simulink model "with_holes"  (R2020b)
settings: Solver=ode23s  StartTime=0.0  StopTime=25  FixedStep=0.2  RelTol=1e-3
PreLoadFcn:
  | sm_tread_drive_param
  | 
  | fuzzy
values from neighbouring files (symbols this model uses):
  ground_x = 12    [sm_tread_drive_param.m]
  ground_y = 10    [sm_tread_drive_param.m]
  tread_l = 2.8    [sm_tread_drive_param.m]
  tread_rad = tread_roller_rad*1.05    (= 0.294)    [sm_tread_drive_param.m]
  tread_roller_rad = tread_h/2*0.8    (= 0.28)    [sm_tread_drive_param.m]
  tread_sep = 1.8    [sm_tread_drive_param.m]
undefined symbols (not defined in the file or in its folder): Extr_Data_RectangleRounded_Holes, floor_d, floor_l, X, Y, Z
libraries: sm_lib x75, nesl_utility x7, Contact_Forces_Lib x6, Parts_Lib x5, fl_lib x4, dspswit3 x1, fuzblock x1, eeGeneralControl x1
(part 1 of 3)
settings Model: Creator=Mario Faragalla  LastModifiedBy=Mario Faragalla
settings DiagnosticsConfigSet: SimMechanicsRigidlyBoundBlock=none

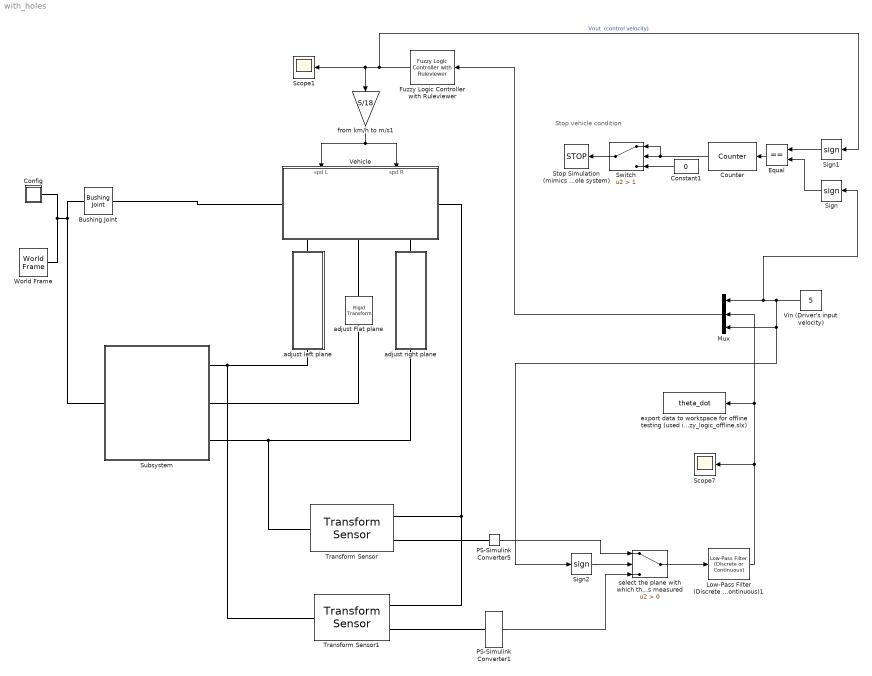
== system with_holes ==
  note: Stop vehicle condition
  Bushing Joint : sm_lib/Joints/Bushing Joint  JointMode=Normal  SenseConstraintForce=off  SenseConstraintForceX=off  SenseConstraintForceY=off  SenseConstraintForceZ=off  SenseConstraintTorque=off  SenseConstraintTorqueX=off  SenseConstraintTorqueY=off  SenseConstraintTorqueZ=off  SenseTotalForce=off  SenseTotalForceX=off  SenseTotalForceY=off  SenseTotalForceZ=off  SenseTotalTorque=off  SenseTotalTorqueX=off  SenseTotalTorqueY=off  SenseTotalTorqueZ=off  CompositeWrenchDir=FollowerOnBase  CompositeWrenchFrame=BaseFrame  PxEquilibriumPosition=0  PxEquilibriumPositionUnits=m  PxSpringStiffness=0  PxSpringStiffnessUnits=N/m  PxDampingCoefficient=0  PxDampingCoefficientUnits=N/(m/s)  PxTorqueActuationMode=NoTorque  PxMotionActuationMode=ComputedMotion  PxSensePosition=off  PxSenseVelocity=off  PxSenseAcceleration=off  PxSenseTorqueForce=off  PxSenseLowerLimitTorqueForce=off  PxSenseUpperLimitTorqueForce=off  PxLowerLimitSpecify=off  PxLowerLimitBound=-1  PxLowerLimitBoundUnits=m  PxLowerLimitStiffness=1e6  PxLowerLimitStiffnessUnits=N/m  PxLowerLimitDamping=1e3  PxLowerLimitDampingUnits=N/(m/s)  PxLowerLimitTransitionRegionWidth=1e-4  PxLowerLimitTransitionRegionWidthUnits=m  PxUpperLimitSpecify=off  PxUpperLimitBound=1  PxUpperLimitBoundUnits=m  PxUpperLimitStiffness=1e6  PxUpperLimitStiffnessUnits=N/m  PxUpperLimitDamping=1e3  PxUpperLimitDampingUnits=N/(m/s)  PxUpperLimitTransitionRegionWidth=1e-4  PxUpperLimitTransitionRegionWidthUnits=m  PxPositionTargetSpecify=on  PxPositionTargetPriority=High  PxPositionTargetValue=-10  PxPositionTargetValueUnits=m  PxVelocityTargetSpecify=off  PxVelocityTargetPriority=High  PxVelocityTargetValue=0  PxVelocityTargetValueUnits=m/s  PyEquilibriumPosition=0  PyEquilibriumPositionUnits=m  PySpringStiffness=0  PySpringStiffnessUnits=N/m  PyDampingCoefficient=0  PyDampingCoefficientUnits=N/(m/s)  PyTorqueActuationMode=NoTorque  PyMotionActuationMode=ComputedMotion  PySensePosition=off  PySenseVelocity=off  PySenseAcceleration=off  PySenseTorqueForce=off  PySenseLowerLimitTorqueForce=off  PySenseUpperLimitTorqueForce=off  PyLowerLimitSpecify=off  PyLowerLimitBound=-1  PyLowerLimitBoundUnits=m  PyLowerLimitStiffness=1e6  PyLowerLimitStiffnessUnits=N/m  PyLowerLimitDamping=1e3  PyLowerLimitDampingUnits=N/(m/s)  PyLowerLimitTransitionRegionWidth=1e-4  PyLowerLimitTransitionRegionWidthUnits=m  PyUpperLimitSpecify=off  PyUpperLimitBound=1  PyUpperLimitBoundUnits=m  PyUpperLimitStiffness=1e6  PyUpperLimitStiffnessUnits=N/m  PyUpperLimitDamping=1e3  PyUpperLimitDampingUnits=N/(m/s)  PyUpperLimitTransitionRegionWidth=1e-4  PyUpperLimitTransitionRegionWidthUnits=m  PyPositionTargetSpecify=on  PyPositionTargetPriority=High  PyPositionTargetValue=0  PyPositionTargetValueUnits=m  PyVelocityTargetSpecify=on  PyVelocityTargetPriority=High  PyVelocityTargetValue=0  PyVelocityTargetValueUnits=m/s  PzEquilibriumPosition=0  PzEquilibriumPositionUnits=m  PzSpringStiffness=0  PzSpringStiffnessUnits=N/m  PzDampingCoefficient=0  PzDampingCoefficientUnits=N/(m/s)  PzTorqueActuationMode=NoTorque  PzMotionActuationMode=ComputedMotion  PzSensePosition=off  PzSenseVelocity=off  PzSenseAcceleration=off  PzSenseTorqueForce=off  PzSenseLowerLimitTorqueForce=off  PzSenseUpperLimitTorqueForce=off  PzLowerLimitSpecify=off  PzLowerLimitBound=-1  PzLowerLimitBoundUnits=m  PzLowerLimitStiffness=1e6  PzLowerLimitStiffnessUnits=N/m  PzLowerLimitDamping=1e3  PzLowerLimitDampingUnits=N/(m/s)  PzLowerLimitTransitionRegionWidth=1e-4  PzLowerLimitTransitionRegionWidthUnits=m  PzUpperLimitSpecify=off  PzUpperLimitBound=1  PzUpperLimitBoundUnits=m  PzUpperLimitStiffness=1e6  PzUpperLimitStiffnessUnits=N/m  PzUpperLimitDamping=1e3  PzUpperLimitDampingUnits=N/(m/s)  PzUpperLimitTransitionRegionWidth=1e-4  PzUpperLimitTransitionRegionWidthUnits=m  PzPositionTargetSpecify=on  PzPositionTargetPriority=High  PzPositionTargetValue=(tread_rad *2)+0.05  PzPositionTargetValueUnits=m  PzVelocityTargetSpecify=off  PzVelocityTargetPriority=High  PzVelocityTargetValue=0  PzVelocityTargetValueUnits=m/s  RxEquilibriumPosition=0  RxEquilibriumPositionUnits=deg  RxSpringStiffness=0  RxSpringStiffnessUnits=N*m/deg  RxDampingCoefficient=0  RxDampingCoefficientUnits=N*m/(deg/s)  RxTorqueActuationMode=NoTorque  RxMotionActuationMode=ComputedMotion  RxSensePosition=off  RxSenseVelocity=off  RxSenseAcceleration=off  RxSenseTorqueForce=off  RxSenseLowerLimitTorqueForce=off  RxSenseUpperLimitTorqueForce=off  RxLowerLimitSpecify=off  RxLowerLimitBound=-90  RxLowerLimitBoundUnits=deg  RxLowerLimitStiffness=1e4  RxLowerLimitStiffnessUnits=N*m/deg  RxLowerLimitDamping=10  RxLowerLimitDampingUnits=N*m/(deg/s)  RxLowerLimitTransitionRegionWidth=0.1  RxLowerLimitTransitionRegionWidthUnits=deg  RxUpperLimitSpecify=off  RxUpperLimitBound=90  RxUpperLimitBoundUnits=deg  RxUpperLimitStiffness=1e4  RxUpperLimitStiffnessUnits=N*m/deg  RxUpperLimitDamping=10  RxUpperLimitDampingUnits=N*m/(deg/s)  RxUpperLimitTransitionRegionWidth=0.1  RxUpperLimitTransitionRegionWidthUnits=deg  RxPositionTargetSpecify=off  RxPositionTargetPriority=High  RxPositionTargetValue=0  RxPositionTargetValueUnits=deg  RxVelocityTargetSpecify=off  RxVelocityTargetPriority=High  RxVelocityTargetValue=0  RxVelocityTargetValueUnits=deg/s  RyEquilibriumPosition=0  RyEquilibriumPositionUnits=deg  RySpringStiffness=0  RySpringStiffnessUnits=N*m/deg  RyDampingCoefficient=0  RyDampingCoefficientUnits=N*m/(deg/s)  RyTorqueActuationMode=NoTorque  RyMotionActuationMode=ComputedMotion  RySensePosition=off  RySenseVelocity=off  RySenseAcceleration=off  RySenseTorqueForce=off  RySenseLowerLimitTorqueForce=off  RySenseUpperLimitTorqueForce=off  RyLowerLimitSpecify=off  RyLowerLimitBound=-90  RyLowerLimitBoundUnits=deg  RyLowerLimitStiffness=1e4  RyLowerLimitStiffnessUnits=N*m/deg  RyLowerLimitDamping=10  RyLowerLimitDampingUnits=N*m/(deg/s)  RyLowerLimitTransitionRegionWidth=0.1  RyLowerLimitTransitionRegionWidthUnits=deg  RyUpperLimitSpecify=off  RyUpperLimitBound=90  RyUpperLimitBoundUnits=deg  RyUpperLimitStiffness=1e4  RyUpperLimitStiffnessUnits=N*m/deg  RyUpperLimitDamping=10  RyUpperLimitDampingUnits=N*m/(deg/s)  RyUpperLimitTransitionRegionWidth=0.1  RyUpperLimitTransitionRegionWidthUnits=deg  RyPositionTargetSpecify=off  RyPositionTargetPriority=High  RyPositionTargetValue=0  RyPositionTargetValueUnits=deg  RyVelocityTargetSpecify=off  RyVelocityTargetPriority=High  RyVelocityTargetValue=0  RyVelocityTargetValueUnits=deg/s  RzEquilibriumPosition=0  RzEquilibriumPositionUnits=deg  RzSpringStiffness=0  RzSpringStiffnessUnits=N*m/deg  RzDampingCoefficient=0  RzDampingCoefficientUnits=N*m/(deg/s)  RzTorqueActuationMode=NoTorque  RzMotionActuationMode=ComputedMotion  RzSensePosition=off  RzSenseVelocity=off  RzSenseAcceleration=off  RzSenseTorqueForce=off  RzSenseLowerLimitTorqueForce=off  RzSenseUpperLimitTorqueForce=off  RzLowerLimitSpecify=off  RzLowerLimitBound=-90  RzLowerLimitBoundUnits=deg  RzLowerLimitStiffness=1e4  RzLowerLimitStiffnessUnits=N*m/deg  RzLowerLimitDamping=10  RzLowerLimitDampingUnits=N*m/(deg/s)  RzLowerLimitTransitionRegionWidth=0.1  RzLowerLimitTransitionRegionWidthUnits=deg  RzUpperLimitSpecify=off  RzUpperLimitBound=90  RzUpperLimitBoundUnits=deg  RzUpperLimitStiffness=1e4  RzUpperLimitStiffnessUnits=N*m/deg  RzUpperLimitDamping=10  RzUpperLimitDampingUnits=N*m/(deg/s)  RzUpperLimitTransitionRegionWidth=0.1  RzUpperLimitTransitionRegionWidthUnits=deg  RzPositionTargetSpecify=off  RzPositionTargetPriority=High  RzPositionTargetValue=0  RzPositionTargetValueUnits=deg  RzVelocityTargetSpecify=off  RzVelocityTargetPriority=High  RzVelocityTargetValue=0  RzVelocityTargetValueUnits=deg/s
  Config : Subsystem
  Constant1 : Constant  Value=0
  Counter : dspswit3/Counter  Direction=Up  CountEvent=Falling edge  CounterSize=User defined  MaxCount=255  InitialCount=0  Output=Count  HitValue=32  ResetInput=off  SamplesPerFrame=1  Ts=1  CntDtype=double  HitDtype=Logical
  Equal : RelationalOperator  Operator===  OutDataTypeStr=boolean  RndMeth=Simplest
  Fuzzy Logic Controller with Ruleviewer : fuzblock/Fuzzy Logic  Controller  with Ruleviewer  fismatrix=fuzzy_pile3  Ts=1
  Low-Pass Filter (Discrete or Continuous)1 : eeGeneralControl/Low-Pass Filter (Discrete or Continuous)  K=10  T=10  B=inf  A=-inf  init_option=Inherited from block input  x0=0  Ts=-1
  Mux : Mux  Inputs=3
  PS-Simulink Converter1 : nesl_utility/PS-Simulink Converter  PhysicalDomain=network_engine_domain  SubClassName=ps_output  LeftPortType=input  RightPortType=output  PseudoPeriodic=off  Frequencies=[]  Unit=inherit  AffineConversion=off
  PS-Simulink Converter5 : nesl_utility/PS-Simulink Converter  PhysicalDomain=network_engine_domain  SubClassName=ps_output  LeftPortType=input  RightPortType=output  PseudoPeriodic=off  Frequencies=[]  Unit=inherit  AffineConversion=off
  Scope1 : Scope
  Scope7 : Scope
  Sign : Signum
  Sign1 : Signum
  Sign2 : Signum
  Stop Simulation (mimics the stop/halt of the whole system) : Stop
  Subsystem : Subsystem
  Switch : Switch  Criteria=u2 > Threshold  Threshold=1  ZeroCross=off
  Transform Sensor : sm_lib/Frames and Transforms/Transform Sensor  MeasurementFrame=Base  SenseAngle=off  SenseAxis=off  SenseAngle1=off  SenseAngle2=off  SenseAngle3=off  SenseQ=off  SenseR=off  SenseOmegaX=off  SenseOmegaY=on  SenseOmegaZ=off  SenseOmega1=off  SenseOmega2=off  SenseOmega3=off  SenseQDot=off  SenseRDot=off  SenseAlphaX=off  SenseAlphaY=off  SenseAlphaZ=off  SenseAlpha1=off  SenseAlpha2=off  SenseAlpha3=off  SenseQDDot=off  SenseRDDot=off  SenseX=off  SenseY=off  SenseZ=off  SenseRad=off  SenseAzim=off  SenseDist=off  SenseInc=off  SenseXDot=off  SenseYDot=off  SenseZDot=off  SenseRadDot=off  SenseAzimDot=off  SenseDistDot=off  SenseIncDot=off  SenseXDDot=off  SenseYDDot=off  SenseZDDot=off  SenseRadDDot=off  SenseAzimDDot=off  SenseDistDDot=off  SenseIncDDot=off
  Transform Sensor1 : sm_lib/Frames and Transforms/Transform Sensor  MeasurementFrame=Base  SenseAngle=off  SenseAxis=off  SenseAngle1=off  SenseAngle2=off  SenseAngle3=off  SenseQ=off  SenseR=off  SenseOmegaX=off  SenseOmegaY=on  SenseOmegaZ=off  SenseOmega1=off  SenseOmega2=off  SenseOmega3=off  SenseQDot=off  SenseRDot=off  SenseAlphaX=off  SenseAlphaY=off  SenseAlphaZ=off  SenseAlpha1=off  SenseAlpha2=off  SenseAlpha3=off  SenseQDDot=off  SenseRDDot=off  SenseX=off  SenseY=off  SenseZ=off  SenseRad=off  SenseAzim=off  SenseDist=off  SenseInc=off  SenseXDot=off  SenseYDot=off  SenseZDot=off  SenseRadDot=off  SenseAzimDot=off  SenseDistDot=off  SenseIncDot=off  SenseXDDot=off  SenseYDDot=off  SenseZDDot=off  SenseRadDDot=off  SenseAzimDDot=off  SenseDistDDot=off  SenseIncDDot=off
  Vehicle : Subsystem
      settings: PortSchema="{\"entries\":[{\"content\":{\"sides\":[{\"content\":{\"connectorIds\":[\"LConn1\"]},\"type\":\"ConnectorPlacement.EquallySpacedRectSide\",\"uuid\":\"fabd707b-f59e-4d45-9dad-4545376ba824\"},{\"content\":{\"connectorIds\":[\"RConn1\"],\"side\":\"RIGHT\"},\"type\":\"ConnectorPlacement.EquallySpacedRectSide\",\"uuid\":\"43ada801-dfb5-4da2-9ab6-aa6db2d15a3d\"},{\"content\":{\"connectorIds\":[\"In1\",\"In2\"],\"side\":\"TOP\"},\"type\":\"ConnectorPlacement.EquallySpacedRectSide\",\"uuid\":\"d91eeb3e-32db-47be-89ab-731665e820f4\"},{\"content\":{\"connectorIds\":[\"RConn2\",\"RConn3\",\"RConn4\"],\"side\":\"BOTTOM\"},\"type\":\"ConnectorPlacement.EquallySpacedRectSide\",\"uuid\":\"76da0d23-ddc9-40dc-a786-2b5b64db7456\"},{\"content\":{\"connectorIds\":[],\"side\":\"HIDDEN\"},\"type\":\"ConnectorPlacement.EquallySpacedRectSide\",\"uuid\":\"48004759-c8c6-47b3-a548-5f1511dff9b7\"}]},\"type\":\"ConnectorPlacement.EquallySpacedConnector\",\"uuid\":\"00c001d2-b8fc-42af-bb12-1d4013db9b0f\"}],\"packageUris\":[\"http://schema.mathworks.com/mf0/Connector/R2020b\"],\"version\":\"1.0\"}"
  Vin (Driver's input velocity) : Constant  Value=5
  World Frame : sm_lib/Frames and Transforms/World Frame
  adjust Flat plane : sm_lib/Frames and Transforms/Rigid Transform  TranslationMethod=StandardAxis  TranslationStandardOffset=(ground_y/4)-0.25  TranslationLengthUnit=m  TranslationStandardAxis=-Y  TranslationCartesianOffset=[0 0 0]  TranslationROffset=0  TranslationROffsetUnits=m  TranslationZOffset=0  TranslationZOffsetUnits=m  TranslationThetaOffset=0  TranslationThetaOffsetUnits=deg  RotationMethod=None  RotationAngleUnits=deg  RotationStandardAxis=+Z  RotationAngle=0.0  RotationArbitraryAxis=[0 0 1]  FollAlignAxisA=+X  BaseAlignAxisA=+Y  FollAlignAxisB=+Y  BaseAlignAxisB=+Z  RotationSequenceAxes=FollowerAxes  RotationSequence=XYX  RotationSequenceAngles=[0 0 0]  RotationSequenceAnglesUnits=deg  RotationMatrix=[1 0 0; 0 1 0; 0 0 1]
  adjust left plane : Subsystem  mask{theta_y=0, offset=up}
      mask prompts: theta_y "Rotation angle"; offset "Direction"
      mask init:
      | switch offset
      |     case 1 %up
      |         offset = -1;
      |     case 2 %down
      |         offset = 1;
      | end
      settings: PortSchema="{\"entries\":[{\"content\":{\"sides\":[{\"content\":{\"connectorIds\":[]},\"type\":\"ConnectorPlacement.EquallySpacedRectSide\",\"uuid\":\"5a52d3ef-8c7d-4b27-92b4-2598d60e8078\"},{\"content\":{\"connectorIds\":[],\"side\":\"RIGHT\"},\"type\":\"ConnectorPlacement.EquallySpacedRectSide\",\"uuid\":\"b8857e3b-9921-4182-868b-79d7343a5054\"},{\"content\":{\"connectorIds\":[\"LConn1\"],\"side\":\"TOP\"},\"type\":\"ConnectorPlacement.EquallySpacedRectSide\",\"uuid\":\"f0e6d2e1-14ee-4037-93b2-310d29a56d19\"},{\"content\":{\"connectorIds\":[\"RConn1\"],\"side\":\"BOTTOM\"},\"type\":\"ConnectorPlacement.EquallySpacedRectSide\",\"uuid\":\"43a24530-94b3-4087-a619-828f9720b0aa\"},{\"content\":{\"connectorIds\":[],\"side\":\"HIDDEN\"},\"type\":\"ConnectorPlacement.EquallySpacedRectSide\",\"uuid\":\"5c2e012c-30d9-4d31-97bb-8e423c4954f3\"}]},\"type\":\"ConnectorPlacement.EquallySpacedConnector\",\"uuid\":\"691960ed-2049-457f-8a6b-8196be0b7b83\"}],\"packageUris\":[\"http://schema.mathworks.com/mf0/Connector/R2020b\"],\"version\":\"1.0\"}"
      mask TypeOptions offset: up | down
  adjust right plane : Subsystem  mask{theta_y=0, offset=down}
      mask prompts: theta_y "Rotation angle"; offset "Direction"
      mask init:
      | switch offset
      |     case 1 %up
      |         offset = 360;
      |     case 2 %down
      |         offset = 2*theta_y;
      | end
      settings: PortSchema="{\"entries\":[{\"content\":{\"sides\":[{\"content\":{\"connectorIds\":[]},\"type\":\"ConnectorPlacement.EquallySpacedRectSide\",\"uuid\":\"5a52d3ef-8c7d-4b27-92b4-2598d60e8078\"},{\"content\":{\"connectorIds\":[],\"side\":\"RIGHT\"},\"type\":\"ConnectorPlacement.EquallySpacedRectSide\",\"uuid\":\"b8857e3b-9921-4182-868b-79d7343a5054\"},{\"content\":{\"connectorIds\":[\"LConn1\"],\"side\":\"TOP\"},\"type\":\"ConnectorPlacement.EquallySpacedRectSide\",\"uuid\":\"f0e6d2e1-14ee-4037-93b2-310d29a56d19\"},{\"content\":{\"connectorIds\":[\"RConn1\"],\"side\":\"BOTTOM\"},\"type\":\"ConnectorPlacement.EquallySpacedRectSide\",\"uuid\":\"43a24530-94b3-4087-a619-828f9720b0aa\"},{\"content\":{\"connectorIds\":[],\"side\":\"HIDDEN\"},\"type\":\"ConnectorPlacement.EquallySpacedRectSide\",\"uuid\":\"5c2e012c-30d9-4d31-97bb-8e423c4954f3\"}]},\"type\":\"ConnectorPlacement.EquallySpacedConnector\",\"uuid\":\"691960ed-2049-457f-8a6b-8196be0b7b83\"}],\"packageUris\":[\"http://schema.mathworks.com/mf0/Connector/R2020b\"],\"version\":\"1.0\"}"
      mask TypeOptions offset: up | down
  export data to workspace for offline testing (used in Test_fuzzy_logic_offline.slx) : ToWorkspace  VariableName=theta_dot  SaveFormat=Timeseries  SampleTime=0.2
  from km/h to m/s1 : Gain  Gain=5/18
  select the plane with which the rotation is measured : Switch  Criteria=u2 > Threshold
  wires:
  from km/h to m/s1/1 -> Vehicle/1(spd L), Vehicle/2(spd R)
  Mux/1 -> Fuzzy Logic Controller with Ruleviewer/1
  Sign/1 -> Equal/2
  Sign1/1 -> Equal/1
  Equal/1 -> Counter/1
  Counter/1 -> Switch/1, Switch/2
  Switch/1 -> Stop Simulation (mimics the stop/halt of the whole system)/1
  Constant1/1 -> Switch/3
  Vin (Driver's input velocity)/1 -> Sign2/1, Mux/3, Mux/1, Sign/1
  Fuzzy Logic Controller with Ruleviewer/1 -> Sign1/1, from km/h to m/s1/1, Scope1/1  "Vout  (control velocity)"
  Sign2/1 -> select the plane with which the rotation is measured/2
  select the plane with which the rotation is measured/1 -> Low-Pass Filter (Discrete or Continuous)1/1
  Low-Pass Filter (Discrete or Continuous)1/1 -> export data to workspace for offline testing (used in Test_fuzzy_logic_offline.slx)/1, Mux/2, Scope7/1
  PS-Simulink Converter5/1 -> select the plane with which the rotation is measured/1
  PS-Simulink Converter1/1 -> select the plane with which the rotation is measured/3
  connections:
  World Frame/RConn1 -- Subsystem/RConn1 -- Bushing Joint/LConn1 -- Config/RConn1
  Vehicle/LConn1 -- Bushing Joint/RConn1
  adjust Flat plane/LConn1 -- Vehicle/RConn3
  Subsystem/LConn1 -- adjust left plane/RConn1 -- Transform Sensor1/LConn1
  Vehicle/RConn1 -- Transform Sensor1/RConn1 -- Transform Sensor/RConn1
  PS-Simulink Converter5/LConn1 -- Transform Sensor/RConn2
  Subsystem/LConn2 -- adjust Flat plane/RConn1
  adjust left plane/LConn1 -- Vehicle/RConn2
  Subsystem/LConn3 -- Transform Sensor/LConn1 -- adjust right plane/RConn1
  adjust right plane/LConn1 -- Vehicle/RConn4
  PS-Simulink Converter1/LConn1 -- Transform Sensor1/RConn2

== system with_holes/Config ==
  Floor : sm_lib/Body Elements/Brick Solid  Commented=on  GraphicAmbientColor=[0.15 0.15 0.15 1.0]  BasedOnType=Density  BrickDimensions=[floor_l floor_l floor_d]  BrickDimensionUnits=m  CenterOfMass=[0 0 0]  CenterOfMassUnits=m  GraphicDiffuseColor=[0.8 0.8 0.8]  Density=1000  DensityUnits=kg/m^3  DoExposeReferenceFrame=on  GraphicEmissiveColor=[0.0 0.0 0.0 1.0]  ExportEntireGeometry=off  SerializedFrames=<Frames><Frame><Id>Frame1</Id><Value><Name>T</Name><Origin><Source>GeometricFeature</Source><FeatureName>+z surface</FeatureName></Origin><PrimaryAxis><DefinedDirection>+Z</DefinedDirection><Source>ReferenceFrame</Source><SourceDirection>+Z</SourceDirection><FeatureName></FeatureName></PrimaryAxis><SecondaryAxis><DefinedDirection>+X</DefinedDirection><Source>ReferenceFrame</Source><SourceDirection>+X</SourceDirection><FeatureName></FeatureName></SecondaryAxis></Value></Frame></Frames>  MarkerShape=Sphere  MarkerSize=10  GraphicType=FromGeometry  InertiaType=CalculateFromGeometry  Mass=1  MassUnits=kg  MomentsOfInertia=[1 1 1]  MomentsOfInertiaUnits=kg*m^2  GraphicOpacity=1.0  ProductsOfInertia=[1 1 1]  ProductsOfInertiaUnits=kg*m^2  GraphicShininess=75  GraphicSpecularColor=[0.5 0.5 0.5 1.0]  GraphicVisPropType=SimpleVisualProperties
  Mechanism Configuration : sm_lib/Utilities/Mechanism Configuration  UniformGravity=Constant  GravityVector=[0 0 -9.80665]  GravityVectorUnits=m/s^2  GravityUnits=m/s^2  LinearizationDelta=0.001  JointModeTransitionNonlinearIterations=2
  Solver Configuration : nesl_utility/Solver Configuration  PhysicalDomain=network_engine_domain  SubClassName=solver  LeftPortType=input  RightPortType=generic  Tones=[]  Harmonics=[]  SimulateNoise=off  Profile=off  UseLocalSampling=off  EnableSwitchedLinearOptims=on  FrequencyDomain=off  UseCCode=off  RelTol=0.001  AbsTol=1e-06  MinStep=1e-09  ToWorkspace=off  RevertToSquareIcSolve=off  NumHomotopyIterations=100  PhasorMode=off  PhasorModeNumHarmonics=1  DoDC=off  ResidualTolerance=1e-09  UseLocalSolver=off  LocalSolverChoice=NE_BACKWARD_EULER_ADVANCER  LocalSolverSampleTime=0.001  DoFixedCost=off  MaxNonlinIter=3  MaxModeIter=2  ComputeImpulses=off  ImpulseIterations=2  LinearAlgebra=Sparse  EquationFormulation=NE_TIME_EF  DelaysMemoryBudget=1024  AutomaticFiltering=on  FilteringTimeConstant=0.001  PartitionStorageMethod=AS_NEEDED  PartitionMemoryBudget=1024  PartitionMethod=FAST
  C : PMIOPort  Side=Right
  connections:
  C/RConn1 -- Floor/LConn1 -- Solver Configuration/RConn1 -- Mechanism Configuration/RConn1

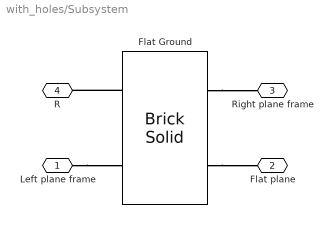
== system with_holes/Subsystem ==
  Flat Ground : sm_lib/Body Elements/Brick Solid  GraphicAmbientColor=[0.15 0.15 0.15 1.0]  BasedOnType=Density  BrickDimensions=[ground_x-3 ground_y 0.5]  BrickDimensionUnits=m  CenterOfMass=[0 0 0]  CenterOfMassUnits=m  GraphicDiffuseColor=[0.5 0.5 0.5]  Density=1000  DensityUnits=kg/m^3  DoExposeReferenceFrame=on  GraphicEmissiveColor=[0.0 0.0 0.0 1.0]  ExportEntireGeometry=off  SerializedFrames=<Frames><Frame><Id>Frame1</Id><Value><Name>F1</Name><Origin><Source>GeometricFeature</Source><FeatureName>-x surface</FeatureName></Origin><PrimaryAxis><DefinedDirection>+Z</DefinedDirection><Source>ReferenceFrame</Source><SourceDirection>+Z</SourceDirection><FeatureName></FeatureName></PrimaryAxis><SecondaryAxis><DefinedDirection>+X</DefinedDirection><Source>ReferenceFrame</Source><SourceDirection>+X</SourceDirection><FeatureName></FeatureName></SecondaryAxis></Value></Frame><Frame><Id>Frame2</Id><Value><Name>Contact F</Name><Origin><Source>CenterOfMassFrame</Source><FeatureName></FeatureName></Origin><PrimaryAxis><DefinedDirection>+Z</DefinedDirection><Source>ReferenceFrame</Source><SourceDirection>+Y</SourceDirection><FeatureName></FeatureName></PrimaryAxis><SecondaryAxis><DefinedDirection>+X</DefinedDirection><Source>ReferenceFrame</Source><SourceDirection>+X</SourceDirection><FeatureName></FeatureName></SecondaryAxis></Value></Frame><Frame><Id>Frame3</Id><Value><Name>F2</Name><Origin><Source>GeometricFeature</Source><FeatureName>+x surface</FeatureName></Origin><PrimaryAxis><DefinedDirection>+Z</DefinedDirection><Source>ReferenceFrame</Source><SourceDirection>+Z</SourceDirection><FeatureName></FeatureName></PrimaryAxis><SecondaryAxis><DefinedDirection>+X</DefinedDirection><Source>ReferenceFrame</Source><SourceDirection>+X</SourceDirection><FeatureName></FeatureName></SecondaryAxis></Value></Frame></Frames>  MarkerShape=Sphere  MarkerSize=10  GraphicType=FromGeometry  InertiaType=CalculateFromGeometry  Mass=1  MassUnits=kg  MomentsOfInertia=[1 1 1]  MomentsOfInertiaUnits=kg*m^2  GraphicOpacity=1.0  ProductsOfInertia=[0 0 0]  ProductsOfInertiaUnits=kg*m^2  GraphicShininess=75  GraphicSpecularColor=[0.5 0.5 0.5 1.0]  GraphicVisPropType=SimpleVisualProperties
  Left plane frame : PMIOPort  Side=Left
  Flat plane : PMIOPort  Port=2  Side=Left
  Right plane frame : PMIOPort  Port=3  Side=Left
  R : PMIOPort  Port=4  Side=Right
  connections:
  Flat Ground/LConn2 -- Flat plane/RConn1
  Flat Ground/RConn1 -- R/RConn1
  Left plane frame/RConn1 -- Flat Ground/RConn2
  Flat Ground/LConn1 -- Right plane frame/RConn1

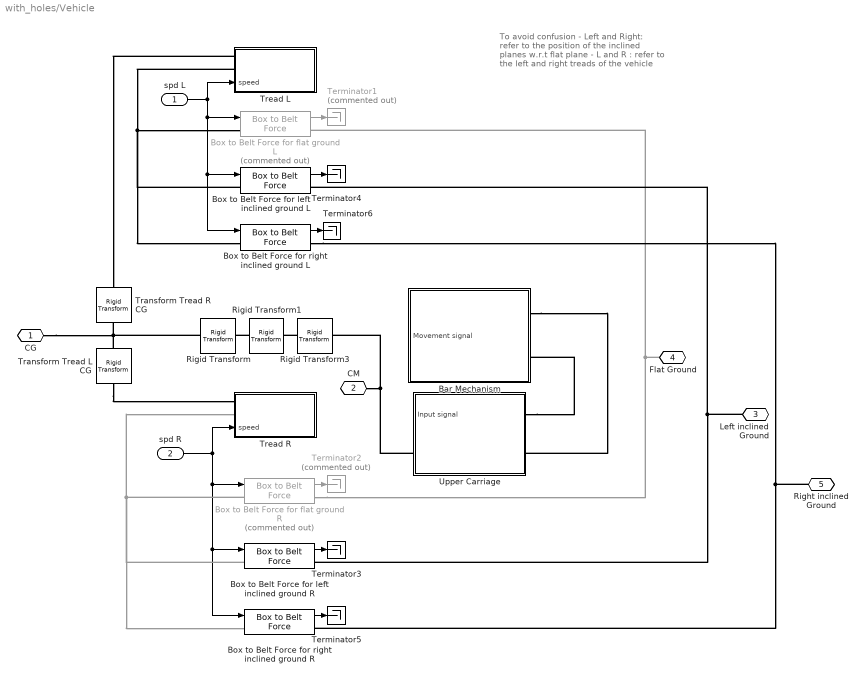
== system with_holes/Vehicle ==
  note: To avoid confusion
      |
      | - Left and Right: refer to the position of the inclined planes w.r.t flat plane
      |
      | - L and R : refer to the left and right treads of the vehicle
  spd L : Inport
  spd R : Inport  Port=2
  Bar Mechanism : Subsystem  mask{barA=3.5, barA1=0.6, trianA=1.2, barB1=1, barB2=0.8, barB3=0.1, barAlpha=80, barA4=0.1, trianR=0.05, barD=0.3, L=0.6, H=0.6, bar_weight=0.8, triangle_weight=1.818, a0=0}
      mask prompts: barA "A1"; barA1 "A2"; trianA "A3"; barB1 "B1"; barB2 "B2"; barB3 "B3"; barAlpha "beta"; barA4 "R1"; trianR "R2"; barD "D"; bar_weight "Bar weight (ton)"; triangle_weight "Triangle weight (ton)"; a0 "alpha"
      mask init:
      | hDistanceBetweenBars = L;
      | vDistanceBetweenBars = H;
      | 
      | barH = (barB1/2-barB2/2)/cosd(barAlpha);
      | barXCoords = [barB1/2,-barB1/2,-barB1/2,-barB1/2+barH*cosd(barAlpha),-barB1/2+barH*cosd(barAlpha),...
      |     barB1/2-barH*cosd(barAlpha),barB1/2-barH*cosd(barAlpha),barB1/2,barB1/2];
      | barYCoords = [barA,barA,barA-barA1,barA-barA1-barH*sind(barAlpha),0,0,barA-barA1-barH*sind(barAlpha),barA-barA1,barA];
      | 
      | barCoords = [barXCoords',barYCoords'];
      | 
      | 
      | barExtraAngle = linspace(0,pi,10);
      | barExtraXCoords = [barD/2,(barD/2)*cos(barExtraAngle),-barD/2];
      | barExtraYCoords = [0,barA1+(barD/2)*sin(barExtraAngle),0];
      | barExtraCoords = [barExtraXCoords',barExtraYCoords'];
      | 
      | 
      | 
      | trianB = sqrt(hDistanceBetweenBars^2+vDistanceBetweenBars^2);
      | %trianA = A;
      | %trianR = 0.05;
      | trianH = sqrt(trianA^2+trianB^2);
      | trianAlpha = 180-atand(trianH/trianR)-atand(trianA/trianB);
      | trianGamma = 90-atand(trianR/trianH)-(90-atand(trianB/trianA));
      | trianXCoords = [trianR*cos(linspace(pi,pi*(3/2),10)),trianB+trianR*cos(linspace(-pi/2,trianAlpha*pi/180,20)),...
      |     trianR*cos(linspace(trianGamma*pi/180,pi,20))];
      |     %,...
      |     %trianR*cos(linspace(pi/3,pi,10))];
      | trianYCoords = [trianR*sin(linspace(pi,pi*(3/2),10)),trianR*sin(linspace(-pi/2,trianAlpha*pi/180,20)),...
      |     trianA+trianR*sin(linspace(trianGamma*pi/180,pi,20))];
      |     %,...
      |     %trianA+trianR*sin(linspace(pi/3,pi,10))];
      | trianCoords = [trianXCoords',trianYCoords'];
      mask DialogControl Container12 Prompt: Dimensions
      mask DialogControl Container11 Prompt: Initial Conditions
      mask Display: image('$imagefile'); % Use "Edit Image" on toolstrip to change.
  Box to Belt Force for flat ground L : Contact_Forces_Lib/2D/Composite Forces/Box to Belt Force  Commented=on  box_l=ground_x-3  box_h=ground_y/2  belt_l=tread_l*1.7  belt_h=(tread_rad+0.1)*2  contact_circle_rad_box2belt=0  force_law_box2belt=Linear  k_contact_box2belt=1e6  b_contact_box2belt=1e5  pen_full_damp_F_box2belt=1e-4  pen_exponent_box2belt=1  friction_law_box2belt=Stick-Slip Continuous  mu_kinetic_box2belt=0.35  mu_static_box2belt=0.4  v_thr_box2belt=0.001  vis_on_box2belt=on  vis_opc_en_box2belt=0  vis_len_boxz=0.1  vis_len_boxx=0.005  vis_len_beltz=0.1  vis_len_beltx=0.005  vis_clr_box2belt=[0 0.2 0.2]  vis_opc_box2belt=0.7
      settings: SourceProductName=Simscape Multibody Contact Forces Library
  Box to Belt Force for flat ground R : Contact_Forces_Lib/2D/Composite Forces/Box to Belt Force  Commented=on  box_l=ground_x-3  box_h=ground_y/2  belt_l=tread_l*1.7  belt_h=(tread_rad+0.1)*2  contact_circle_rad_box2belt=0  force_law_box2belt=Linear  k_contact_box2belt=1e6  b_contact_box2belt=1e5  pen_full_damp_F_box2belt=1e-4  pen_exponent_box2belt=1  friction_law_box2belt=Stick-Slip Continuous  mu_kinetic_box2belt=0.35  mu_static_box2belt=0.4  v_thr_box2belt=0.001  vis_on_box2belt=on  vis_opc_en_box2belt=0  vis_len_boxz=0.1  vis_len_boxx=0.005  vis_len_beltz=0.1  vis_len_beltx=0.005  vis_clr_box2belt=[0 0.2 0.2]  vis_opc_box2belt=0.7
      settings: SourceProductName=Simscape Multibody Contact Forces Library
  Box to Belt Force for left inclined ground L : Contact_Forces_Lib/2D/Composite Forces/Box to Belt Force  box_l=ground_x*2  box_h=ground_y/2  belt_l=tread_l*1.7  belt_h=(tread_rad+0.1)*2  contact_circle_rad_box2belt=0  force_law_box2belt=Linear  k_contact_box2belt=1e6  b_contact_box2belt=1e5  pen_full_damp_F_box2belt=1e-4  pen_exponent_box2belt=1  friction_law_box2belt=Stick-Slip Continuous  mu_kinetic_box2belt=0.35  mu_static_box2belt=0.4  v_thr_box2belt=0.001  vis_on_box2belt=on  vis_opc_en_box2belt=0  vis_len_boxz=0.1  vis_len_boxx=0.005  vis_len_beltz=0.1  vis_len_beltx=0.005  vis_clr_box2belt=[0 0.2 0.2]  vis_opc_box2belt=0.7
      settings: SourceProductName=Simscape Multibody Contact Forces Library
  Box to Belt Force for left inclined ground R : Contact_Forces_Lib/2D/Composite Forces/Box to Belt Force  box_l=ground_x*2  box_h=ground_y/2  belt_l=tread_l*1.7  belt_h=(tread_rad+0.1)*2  contact_circle_rad_box2belt=0  force_law_box2belt=Linear  k_contact_box2belt=1e6  b_contact_box2belt=1e5  pen_full_damp_F_box2belt=1e-4  pen_exponent_box2belt=1  friction_law_box2belt=Stick-Slip Continuous  mu_kinetic_box2belt=0.35  mu_static_box2belt=0.4  v_thr_box2belt=0.001  vis_on_box2belt=on  vis_opc_en_box2belt=0  vis_len_boxz=0.1  vis_len_boxx=0.005  vis_len_beltz=0.1  vis_len_beltx=0.005  vis_clr_box2belt=[0 0.2 0.2]  vis_opc_box2belt=0.7
      settings: SourceProductName=Simscape Multibody Contact Forces Library
  Box to Belt Force for right inclined ground L : Contact_Forces_Lib/2D/Composite Forces/Box to Belt Force  box_l=ground_x*2  box_h=ground_y/2  belt_l=tread_l*1.7  belt_h=(tread_rad+0.1)*2  contact_circle_rad_box2belt=0  force_law_box2belt=Linear  k_contact_box2belt=1e6  b_contact_box2belt=1e5  pen_full_damp_F_box2belt=1e-4  pen_exponent_box2belt=1  friction_law_box2belt=Stick-Slip Continuous  mu_kinetic_box2belt=0.35  mu_static_box2belt=0.4  v_thr_box2belt=0.001  vis_on_box2belt=on  vis_opc_en_box2belt=0  vis_len_boxz=0.1  vis_len_boxx=0.005  vis_len_beltz=0.1  vis_len_beltx=0.005  vis_clr_box2belt=[0 0.2 0.2]  vis_opc_box2belt=0.7
      settings: SourceProductName=Simscape Multibody Contact Forces Library
  Box to Belt Force for right inclined ground R : Contact_Forces_Lib/2D/Composite Forces/Box to Belt Force  box_l=ground_x*2  box_h=ground_y/2  belt_l=tread_l*1.7  belt_h=(tread_rad+0.1)*2  contact_circle_rad_box2belt=0  force_law_box2belt=Linear  k_contact_box2belt=1e6  b_contact_box2belt=1e5  pen_full_damp_F_box2belt=1e-4  pen_exponent_box2belt=1  friction_law_box2belt=Stick-Slip Continuous  mu_kinetic_box2belt=0.35  mu_static_box2belt=0.4  v_thr_box2belt=0.001  vis_on_box2belt=on  vis_opc_en_box2belt=0  vis_len_boxz=0.1  vis_len_boxx=0.005  vis_len_beltz=0.1  vis_len_beltx=0.005  vis_clr_box2belt=[0 0.2 0.2]  vis_opc_box2belt=0.7
      settings: SourceProductName=Simscape Multibody Contact Forces Library
  Rigid Transform : sm_lib/Frames and Transforms/Rigid Transform  TranslationMethod=StandardAxis  TranslationStandardOffset=0.7  TranslationLengthUnit=m  TranslationStandardAxis=-Z  TranslationCartesianOffset=[0 0 0]  TranslationROffset=0  TranslationROffsetUnits=m  TranslationZOffset=0  TranslationZOffsetUnits=m  TranslationThetaOffset=0  TranslationThetaOffsetUnits=deg  RotationMethod=None  RotationAngleUnits=deg  RotationStandardAxis=+Z  RotationAngle=0.0  RotationArbitraryAxis=[0 0 1]  FollAlignAxisA=+X  BaseAlignAxisA=+Y  FollAlignAxisB=+Y  BaseAlignAxisB=+Z  RotationSequenceAxes=FollowerAxes  RotationSequence=XYX  RotationSequenceAngles=[0 0 0]  RotationSequenceAnglesUnits=deg  RotationMatrix=[1 0 0; 0 1 0; 0 0 1]
  Rigid Transform1 : sm_lib/Frames and Transforms/Rigid Transform  TranslationMethod=StandardAxis  TranslationStandardOffset=-2  TranslationLengthUnit=m  TranslationStandardAxis=+X  TranslationCartesianOffset=[0 0 0]  TranslationROffset=0  TranslationROffsetUnits=m  TranslationZOffset=0  TranslationZOffsetUnits=m  TranslationThetaOffset=0  TranslationThetaOffsetUnits=deg  RotationMethod=None  RotationAngleUnits=deg  RotationStandardAxis=+Z  RotationAngle=0.0  RotationArbitraryAxis=[0 0 1]  FollAlignAxisA=+X  BaseAlignAxisA=+Y  FollAlignAxisB=+Y  BaseAlignAxisB=+Z  RotationSequenceAxes=FollowerAxes  RotationSequence=XYX  RotationSequenceAngles=[0 0 0]  RotationSequenceAnglesUnits=deg  RotationMatrix=[1 0 0; 0 1 0; 0 0 1]
  Rigid Transform3 : sm_lib/Frames and Transforms/Rigid Transform  TranslationMethod=StandardAxis  TranslationStandardOffset=0.1  TranslationLengthUnit=m  TranslationStandardAxis=+Y  TranslationCartesianOffset=[0 0 0]  TranslationROffset=0  TranslationROffsetUnits=m  TranslationZOffset=0  TranslationZOffsetUnits=m  TranslationThetaOffset=0  TranslationThetaOffsetUnits=deg  RotationMethod=None  RotationAngleUnits=deg  RotationStandardAxis=+Z  RotationAngle=0.0  RotationArbitraryAxis=[0 0 1]  FollAlignAxisA=+X  BaseAlignAxisA=+Y  FollAlignAxisB=+Y  BaseAlignAxisB=+Z  RotationSequenceAxes=FollowerAxes  RotationSequence=XYX  RotationSequenceAngles=[0 0 0]  RotationSequenceAnglesUnits=deg  RotationMatrix=[1 0 0; 0 1 0; 0 0 1]
  Terminator1 : Terminator  Commented=on
  Terminator2 : Terminator  Commented=on
  Terminator{3..6} (4 alike) : Terminator
  Transform Tread L CG : sm_lib/Frames and Transforms/Rigid Transform  TranslationMethod=StandardAxis  TranslationStandardOffset=tread_sep/2  TranslationLengthUnit=m  TranslationStandardAxis=+Y  TranslationCartesianOffset=[0 0 0]  TranslationROffset=0  TranslationROffsetUnits=m  TranslationZOffset=0  TranslationZOffsetUnits=m  TranslationThetaOffset=0  TranslationThetaOffsetUnits=deg  RotationMethod=None  RotationAngleUnits=deg  RotationStandardAxis=+Z  RotationAngle=0.0  RotationArbitraryAxis=[0 0 1]  FollAlignAxisA=+X  BaseAlignAxisA=+Y  FollAlignAxisB=+Y  BaseAlignAxisB=+Z  RotationSequenceAxes=FollowerAxes  RotationSequence=XYX  RotationSequenceAngles=[0 0 0]  RotationSequenceAnglesUnits=deg  RotationMatrix=[1 0 0; 0 1 0; 0 0 1]
  Transform Tread R CG : sm_lib/Frames and Transforms/Rigid Transform  TranslationMethod=StandardAxis  TranslationStandardOffset=tread_sep/2  TranslationLengthUnit=m  TranslationStandardAxis=+Y  TranslationCartesianOffset=[0 0 0]  TranslationROffset=0  TranslationROffsetUnits=m  TranslationZOffset=0  TranslationZOffsetUnits=m  TranslationThetaOffset=0  TranslationThetaOffsetUnits=deg  RotationMethod=None  RotationAngleUnits=deg  RotationStandardAxis=+Z  RotationAngle=0.0  RotationArbitraryAxis=[0 0 1]  FollAlignAxisA=+X  BaseAlignAxisA=+Y  FollAlignAxisB=+Y  BaseAlignAxisB=+Z  RotationSequenceAxes=FollowerAxes  RotationSequence=XYX  RotationSequenceAngles=[0 0 0]  RotationSequenceAnglesUnits=deg  RotationMatrix=[1 0 0; 0 1 0; 0 0 1]
  Tread L : Subsystem
      settings: PortSchema="{\"entries\":[{\"content\":{\"sides\":[{\"content\":{\"connectorIds\":[]},\"type\":\"ConnectorPlacement.EquallySpacedRectSide\",\"uuid\":\"71f54ac7-1acd-4494-b2ba-36120ebb2448\"},{\"content\":{\"connectorIds\":[\"RConn1\",\"RConn2\",\"In1\"],\"side\":\"RIGHT\"},\"type\":\"ConnectorPlacement.EquallySpacedRectSide\",\"uuid\":\"abfaafc8-7934-4bf8-9c1d-7af05f31c6a7\"},{\"content\":{\"connectorIds\":[],\"side\":\"TOP\"},\"type\":\"ConnectorPlacement.EquallySpacedRectSide\",\"uuid\":\"b5262782-7ab0-48f5-b129-0cdfcd7050d8\"},{\"content\":{\"connectorIds\":[],\"side\":\"BOTTOM\"},\"type\":\"ConnectorPlacement.EquallySpacedRectSide\",\"uuid\":\"5c554a08-2f46-428a-a953-6231f81c923d\"},{\"content\":{\"connectorIds\":[],\"side\":\"HIDDEN\"},\"type\":\"ConnectorPlacement.EquallySpacedRectSide\",\"uuid\":\"0cc664ae-e858-4ab8-8762-0f97b2d06f3c\"}]},\"type\":\"ConnectorPlacement.EquallySpacedConnector\",\"uuid\":\"cf0c008a-5e1f-4cc9-b20e-5a159a9bbf66\"}],\"packageUris\":[\"http://schema.mathworks.com/mf0/Connector/R2020b\"],\"version\":\"1.0\"}"
  Tread R : Subsystem
      settings: PortSchema="{\"entries\":[{\"content\":{\"sides\":[{\"content\":{\"connectorIds\":[]},\"type\":\"ConnectorPlacement.EquallySpacedRectSide\",\"uuid\":\"71f54ac7-1acd-4494-b2ba-36120ebb2448\"},{\"content\":{\"connectorIds\":[\"RConn1\",\"RConn2\",\"In1\"],\"side\":\"RIGHT\"},\"type\":\"ConnectorPlacement.EquallySpacedRectSide\",\"uuid\":\"abfaafc8-7934-4bf8-9c1d-7af05f31c6a7\"},{\"content\":{\"connectorIds\":[],\"side\":\"TOP\"},\"type\":\"ConnectorPlacement.EquallySpacedRectSide\",\"uuid\":\"b5262782-7ab0-48f5-b129-0cdfcd7050d8\"},{\"content\":{\"connectorIds\":[],\"side\":\"HIDDEN\"},\"type\":\"ConnectorPlacement.EquallySpacedRectSide\",\"uuid\":\"0cc664ae-e858-4ab8-8762-0f97b2d06f3c\"}]},\"type\":\"ConnectorPlacement.EquallySpacedConnector\",\"uuid\":\"cf0c008a-5e1f-4cc9-b20e-5a159a9bbf66\"}],\"packageUris\":[\"http://schema.mathworks.com/mf0/Connector/R2020b\"],\"version\":\"1.0\"}"
  Upper Carriage : Subsystem  mask{A1=2.87, A2=2.725, A3=3.5, B1=2.8, B2=1.12, B3=0.81, B4=1.845, B5=2.8/2, C1=2.196, CW=11, CCW=10, H=0.6, L=0.6}
      mask prompts: CW "Car Weight (ton)"; CCW "Counter Weight Weight (ton)"; H "H*"; L "L*"
      mask init:
      | counterWeightLength = B3;
      | carLength = A2+A1-counterWeightLength;
      | carWidth = B1;
      | carCabinLength = A2%carLength*0.6;
      | carCabinWidth = B2 %carWidth*0.4;
      | counterWeightWidth = carWidth;
      | carHeight = C1;
      | counterWeightHeight = carHeight;
      | carBarBackX = B4;
      | hDistanceBetweenBars = L;
      | vDistanceBetweenBars = H;
      | %Extrusion in Y
      | carCoordX = [0,0,-carWidth,-carWidth,-carCabinWidth,-carCabinWidth];
      | carCoordY = [0,carLength,carLength,carCabinLength,carCabinLength,0];
      | %plot(carCoordX,carCoordY)
      | 
      | carCoord = [carCoordX',carCoordY'];
      | 
      | counterWeightCoordX = [0,0,-carWidth,-carWidth];
      | counterWeightCoordY = [0,counterWeightLength,counterWeightLength,0];
      | %plot(counterWeightCoordX,counterWeightCoordY)
      | counterWeightCoord = [counterWeightCoordX',counterWeightCoordY'];
      mask DialogControl Control4 Prompt: Connection with bar mechanism
      mask DialogControl Control3 Prompt: H* and L* have to be the same as H and L in bar mechanism
      mask Display: image('$imagefile'); % Use "Edit Image" on toolstrip to change.
  CG : PMIOPort  Side=Left
  CM : PMIOPort  Port=2  Side=Right
  Left inclined Ground : PMIOPort  Port=3  Side=Right
  Flat Ground : PMIOPort  Port=4  Side=Right
  Right inclined Ground : PMIOPort  Port=5  Side=Right
  wires:
  Box to Belt Force for flat ground L/1 -> Terminator1/1
  spd L/1 -> Box to Belt Force for right inclined ground L/1, Box to Belt Force for left inclined ground L/1, Box to Belt Force for flat ground L/1, Tread L/1(speed)
  spd R/1 -> Tread R/1(speed), Box to Belt Force for right inclined ground R/1, Box to Belt Force for left inclined ground R/1, Box to Belt Force for flat ground R/1
  Box to Belt Force for flat ground R/1 -> Terminator2/1
  Box to Belt Force for left inclined ground R/1 -> Terminator3/1
  Box to Belt Force for left inclined ground L/1 -> Terminator4/1
  Box to Belt Force for right inclined ground R/1 -> Terminator5/1
  Box to Belt Force for right inclined ground L/1 -> Terminator6/1
  connections:
  CG/RConn1 -- Rigid Transform/RConn1 -- Transform Tread L CG/LConn1 -- Transform Tread R CG/RConn1
  Transform Tread L CG/RConn1 -- Tread R/RConn1
  Tread L/RConn1 -- Transform Tread R CG/LConn1
  Rigid Transform1/RConn1 -- Rigid Transform/LConn1
  Upper Carriage/LConn1 -- Rigid Transform3/LConn1 -- CM/RConn1
  Upper Carriage/RConn1 -- Bar Mechanism/RConn2
  Bar Mechanism/RConn1 -- Upper Carriage/RConn2
  Rigid Transform3/RConn1 -- Rigid Transform1/LConn1
  Tread L/RConn2 -- Box to Belt Force for left inclined ground L/LConn1 -- Box to Belt Force for right inclined ground L/LConn1 -- Box to Belt Force for flat ground L/LConn1
  Box to Belt Force for flat ground R/RConn1 -- Box to Belt Force for flat ground L/RConn1 -- Flat Ground/RConn1
  Box to Belt Force for flat ground R/LConn1 -- Box to Belt Force for left inclined ground R/LConn1 -- Box to Belt Force for right inclined ground R/LConn1 -- Tread R/RConn2
  Left inclined Ground/RConn1 -- Box to Belt Force for left inclined ground R/RConn1 -- Box to Belt Force for left inclined ground L/RConn1
  Box to Belt Force for right inclined ground L/RConn1 -- Box to Belt Force for right inclined ground R/RConn1 -- Right inclined Ground/RConn1

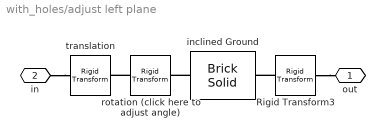
== system with_holes/adjust left plane ==
  Rigid Transform3 : sm_lib/Frames and Transforms/Rigid Transform  TranslationMethod=StandardAxis  TranslationStandardOffset=(ground_y/4)-0.25  TranslationLengthUnit=m  TranslationStandardAxis=+Y  TranslationCartesianOffset=[0 0 0]  TranslationROffset=0  TranslationROffsetUnits=m  TranslationZOffset=0  TranslationZOffsetUnits=m  TranslationThetaOffset=0  TranslationThetaOffsetUnits=deg  RotationMethod=None  RotationAngleUnits=deg  RotationStandardAxis=+Z  RotationAngle=0.0  RotationArbitraryAxis=[0 0 1]  FollAlignAxisA=+X  BaseAlignAxisA=+Y  FollAlignAxisB=+Y  BaseAlignAxisB=+Z  RotationSequenceAxes=FollowerAxes  RotationSequence=XYX  RotationSequenceAngles=[0 0 0]  RotationSequenceAnglesUnits=deg  RotationMatrix=[1 0 0; 0 1 0; 0 0 1]
  inclined Ground : sm_lib/Body Elements/Brick Solid  GraphicAmbientColor=[0.15 0.15 0.15 1.0]  BasedOnType=Density  BrickDimensions=[ground_x*2 ground_y 0.5]  BrickDimensionUnits=m  CenterOfMass=[0 0 0]  CenterOfMassUnits=m  GraphicDiffuseColor=[0.5 0.5 0.5]  Density=1000  DensityUnits=kg/m^3  DoExposeReferenceFrame=off  GraphicEmissiveColor=[0.0 0.0 0.0 1.0]  ExportEntireGeometry=off  SerializedFrames=<Frames><Frame><Id>Frame1</Id><Value><Name>F1</Name><Origin><Source>GeometricFeature</Source><FeatureName>-x surface</FeatureName></Origin><PrimaryAxis><DefinedDirection>+Z</DefinedDirection><Source>ReferenceFrame</Source><SourceDirection>+Z</SourceDirection><FeatureName></FeatureName></PrimaryAxis><SecondaryAxis><DefinedDirection>+X</DefinedDirection><Source>ReferenceFrame</Source><SourceDirection>+X</SourceDirection><FeatureName></FeatureName></SecondaryAxis></Value></Frame><Frame><Id>Frame2</Id><Value><Name>Contact F</Name><Origin><Source>CenterOfMassFrame</Source><FeatureName></FeatureName></Origin><PrimaryAxis><DefinedDirection>+Z</DefinedDirection><Source>ReferenceFrame</Source><SourceDirection>+Y</SourceDirection><FeatureName></FeatureName></PrimaryAxis><SecondaryAxis><DefinedDirection>+X</DefinedDirection><Source>ReferenceFrame</Source><SourceDirection>+X</SourceDirection><FeatureName></FeatureName></SecondaryAxis></Value></Frame></Frames>  MarkerShape=Sphere  MarkerSize=10  GraphicType=FromGeometry  InertiaType=CalculateFromGeometry  Mass=1  MassUnits=kg  MomentsOfInertia=[1 1 1]  MomentsOfInertiaUnits=kg*m^2  GraphicOpacity=1.0  ProductsOfInertia=[0 0 0]  ProductsOfInertiaUnits=kg*m^2  GraphicShininess=75  GraphicSpecularColor=[0.5 0.5 0.5 1.0]  GraphicVisPropType=SimpleVisualProperties
  rotation (click here to adjust angle) : sm_lib/Frames and Transforms/Rigid Transform  TranslationMethod=None  TranslationStandardOffset=0  TranslationLengthUnit=m  TranslationStandardAxis=+Z  TranslationCartesianOffset=[0 0 0]  TranslationROffset=0  TranslationROffsetUnits=m  TranslationZOffset=0  TranslationZOffsetUnits=m  TranslationThetaOffset=0  TranslationThetaOffsetUnits=deg  RotationMethod=StandardAxis  RotationAngleUnits=deg  RotationStandardAxis=+Y  RotationAngle=180-(offset*theta_y)  RotationArbitraryAxis=[0 0 1]  FollAlignAxisA=+X  BaseAlignAxisA=+Y  FollAlignAxisB=+Y  BaseAlignAxisB=+Z  RotationSequenceAxes=FollowerAxes  RotationSequence=XYX  RotationSequenceAngles=[0 0 0]  RotationSequenceAnglesUnits=deg  RotationMatrix=[1 0 0; 0 1 0; 0 0 1]
  translation : sm_lib/Frames and Transforms/Rigid Transform  TranslationMethod=StandardAxis  TranslationStandardOffset=ground_x  TranslationLengthUnit=m  TranslationStandardAxis=-X  TranslationCartesianOffset=[0 0 0]  TranslationROffset=0  TranslationROffsetUnits=m  TranslationZOffset=0  TranslationZOffsetUnits=m  TranslationThetaOffset=0  TranslationThetaOffsetUnits=deg  RotationMethod=None  RotationAngleUnits=deg  RotationStandardAxis=+Y  RotationAngle=45.0  RotationArbitraryAxis=[0 0 1]  FollAlignAxisA=+X  BaseAlignAxisA=+Y  FollAlignAxisB=+Y  BaseAlignAxisB=+Z  RotationSequenceAxes=FollowerAxes  RotationSequence=XYX  RotationSequenceAngles=[0 0 0]  RotationSequenceAnglesUnits=deg  RotationMatrix=[1 0 0; 0 1 0; 0 0 1]
  out : PMIOPort  Side=Left
  in : PMIOPort  Port=2  Side=Right
  connections:
  Rigid Transform3/RConn1 -- inclined Ground/RConn1
  inclined Ground/LConn1 -- rotation (click here to adjust angle)/RConn1
  rotation (click here to adjust angle)/LConn1 -- translation/RConn1
  Rigid Transform3/LConn1 -- out/RConn1
  in/RConn1 -- translation/LConn1

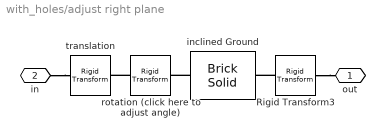
== system with_holes/adjust right plane ==
  Rigid Transform3 : sm_lib/Frames and Transforms/Rigid Transform  TranslationMethod=StandardAxis  TranslationStandardOffset=(ground_y/4)-0.25  TranslationLengthUnit=m  TranslationStandardAxis=-Y  TranslationCartesianOffset=[0 0 0]  TranslationROffset=0  TranslationROffsetUnits=m  TranslationZOffset=0  TranslationZOffsetUnits=m  TranslationThetaOffset=0  TranslationThetaOffsetUnits=deg  RotationMethod=None  RotationAngleUnits=deg  RotationStandardAxis=+Z  RotationAngle=0.0  RotationArbitraryAxis=[0 0 1]  FollAlignAxisA=+X  BaseAlignAxisA=+Y  FollAlignAxisB=+Y  BaseAlignAxisB=+Z  RotationSequenceAxes=FollowerAxes  RotationSequence=XYX  RotationSequenceAngles=[0 0 0]  RotationSequenceAnglesUnits=deg  RotationMatrix=[1 0 0; 0 1 0; 0 0 1]
  inclined Ground : sm_lib/Body Elements/Brick Solid  GraphicAmbientColor=[0.15 0.15 0.15 1.0]  BasedOnType=Density  BrickDimensions=[ground_x*2 ground_y 0.5]  BrickDimensionUnits=m  CenterOfMass=[0 0 0]  CenterOfMassUnits=m  GraphicDiffuseColor=[0.5 0.5 0.5]  Density=1000  DensityUnits=kg/m^3  DoExposeReferenceFrame=off  GraphicEmissiveColor=[0.0 0.0 0.0 1.0]  ExportEntireGeometry=off  SerializedFrames=<Frames><Frame><Id>Frame1</Id><Value><Name>F1</Name><Origin><Source>GeometricFeature</Source><FeatureName>-x surface</FeatureName></Origin><PrimaryAxis><DefinedDirection>+Z</DefinedDirection><Source>ReferenceFrame</Source><SourceDirection>+Z</SourceDirection><FeatureName></FeatureName></PrimaryAxis><SecondaryAxis><DefinedDirection>+X</DefinedDirection><Source>ReferenceFrame</Source><SourceDirection>+X</SourceDirection><FeatureName></FeatureName></SecondaryAxis></Value></Frame><Frame><Id>Frame2</Id><Value><Name>Contact F</Name><Origin><Source>CenterOfMassFrame</Source><FeatureName></FeatureName></Origin><PrimaryAxis><DefinedDirection>+Z</DefinedDirection><Source>ReferenceFrame</Source><SourceDirection>+Y</SourceDirection><FeatureName></FeatureName></PrimaryAxis><SecondaryAxis><DefinedDirection>+X</DefinedDirection><Source>ReferenceFrame</Source><SourceDirection>+X</SourceDirection><FeatureName></FeatureName></SecondaryAxis></Value></Frame></Frames>  MarkerShape=Sphere  MarkerSize=10  GraphicType=FromGeometry  InertiaType=CalculateFromGeometry  Mass=1  MassUnits=kg  MomentsOfInertia=[1 1 1]  MomentsOfInertiaUnits=kg*m^2  GraphicOpacity=1.0  ProductsOfInertia=[0 0 0]  ProductsOfInertiaUnits=kg*m^2  GraphicShininess=75  GraphicSpecularColor=[0.5 0.5 0.5 1.0]  GraphicVisPropType=SimpleVisualProperties
  rotation (click here to adjust angle) : sm_lib/Frames and Transforms/Rigid Transform  TranslationMethod=None  TranslationStandardOffset=0  TranslationLengthUnit=m  TranslationStandardAxis=+Z  TranslationCartesianOffset=[0 0 0]  TranslationROffset=0  TranslationROffsetUnits=m  TranslationZOffset=0  TranslationZOffsetUnits=m  TranslationThetaOffset=0  TranslationThetaOffsetUnits=deg  RotationMethod=StandardAxis  RotationAngleUnits=deg  RotationStandardAxis=+Y  RotationAngle=offset-theta_y  RotationArbitraryAxis=[0 0 1]  FollAlignAxisA=+X  BaseAlignAxisA=+Y  FollAlignAxisB=+Y  BaseAlignAxisB=+Z  RotationSequenceAxes=FollowerAxes  RotationSequence=XYX  RotationSequenceAngles=[0 0 0]  RotationSequenceAnglesUnits=deg  RotationMatrix=[1 0 0; 0 1 0; 0 0 1]
  translation : sm_lib/Frames and Transforms/Rigid Transform  TranslationMethod=StandardAxis  TranslationStandardOffset=ground_x  TranslationLengthUnit=m  TranslationStandardAxis=+X  TranslationCartesianOffset=[0 0 0]  TranslationROffset=0  TranslationROffsetUnits=m  TranslationZOffset=0  TranslationZOffsetUnits=m  TranslationThetaOffset=0  TranslationThetaOffsetUnits=deg  RotationMethod=None  RotationAngleUnits=deg  RotationStandardAxis=+Y  RotationAngle=45.0  RotationArbitraryAxis=[0 0 1]  FollAlignAxisA=+X  BaseAlignAxisA=+Y  FollAlignAxisB=+Y  BaseAlignAxisB=+Z  RotationSequenceAxes=FollowerAxes  RotationSequence=XYX  RotationSequenceAngles=[0 0 0]  RotationSequenceAnglesUnits=deg  RotationMatrix=[1 0 0; 0 1 0; 0 0 1]
  out : PMIOPort  Side=Left
  in : PMIOPort  Port=2  Side=Right
  connections:
  in/RConn1 -- translation/LConn1
  Rigid Transform3/LConn1 -- out/RConn1
  rotation (click here to adjust angle)/LConn1 -- translation/RConn1
  inclined Ground/LConn1 -- rotation (click here to adjust angle)/RConn1
  Rigid Transform3/RConn1 -- inclined Ground/RConn1
